simulink model "parallel_force_pos_control"  (R2020b)
settings: Solver=FixedStepAuto  StartTime=0.0  StopTime=10  FixedStep=Ts  RelTol=1e-3
undefined symbols (not defined in the file): dqi, fd, invMd, K, KD, KF, KI, KP, Md, myRobot, qi, xd, xr
settings Model: Creator=simon  LastModifiedBy=SimoneCremasco
settings SolverCC: ZeroCrossControl=DisableAll

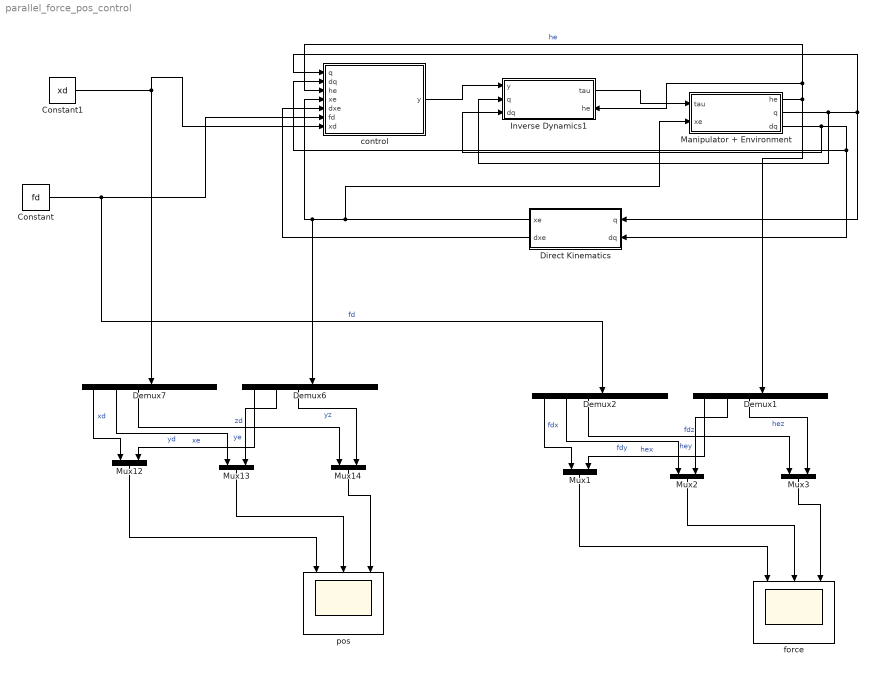
== system parallel_force_pos_control ==
  Constant : Constant  Value=fd
  Constant1 : Constant  Value=xd
  Demux{1..2,6..7} (4 alike) : Demux  Outputs=6
  Direct Kinematics : Subsystem
  Inverse Dynamics1 : Subsystem
      settings: PortSchema="{\"entries\":[{\"content\":{\"sides\":[{\"content\":{\"connectorIds\":[\"In1\",\"In2\",\"In3\"]},\"type\":\"ConnectorPlacement.EquallySpacedRectSide\",\"uuid\":\"75fd2aef-6636-4229-8361-fd4aaeafc71d\"},{\"content\":{\"connectorIds\":[\"Out1\",\"In4\"],\"side\":\"RIGHT\"},\"type\":\"ConnectorPlacement.EquallySpacedRectSide\",\"uuid\":\"1144ef1f-b296-4ded-9ece-76b41f9ae70a\"},{\"content\":{\"connectorIds\":[],\"side\":\"TOP\"},\"type\":\"ConnectorPlacement.EquallySpacedRectSide\",\"uuid\":\"a2369661-a37d-42fa-931f-950a2098898d\"},{\"content\":{\"connectorIds\":[],\"side\":\"BOTTOM\"},\"type\":\"ConnectorPlacement.EquallySpacedRectSide\",\"uuid\":\"99474d0a-a266-4b98-966c-e86b0204795e\"},{\"content\":{\"connectorIds\":[],\"side\":\"HIDDEN\"},\"type\":\"ConnectorPlacement.EquallySpacedRectSide\",\"uuid\":\"b2ea56db-8612-481b-8b10-64691d881ee0\"}]},\"type\":\"ConnectorPlacement.EquallySpacedConnector\",\"uuid\":\"7eb160dc-bfe8-4791-8ee2-e581093abb5e\"}],\"packageUris\":[\"http://schema.mathworks.com/mf0/Connector/R2020b\"],\"version\":\"1.0\"}"
  Manipulator + Environment : Subsystem
  Mux{1..3,12..14} (6 alike) : Mux  Inputs=2
  control : Subsystem
  force : Scope  NumInputPorts=3
  pos : Scope  NumInputPorts=3
  wires:
  Direct Kinematics/2(dxe) -> control/5(dxe)
  control/1(y) -> Inverse Dynamics1/1(y)
  Inverse Dynamics1/1(tau) -> Manipulator + Environment/1(tau)
  Manipulator + Environment/2(q) -> Inverse Dynamics1/2(q), Direct Kinematics/1(q), control/1(q)
  Manipulator + Environment/3(dq) -> Inverse Dynamics1/3(dq), Direct Kinematics/2(dq), control/2(dq)
  Manipulator + Environment/1(he) -> Inverse Dynamics1/4(he), control/3(he), Demux1/1  "he"
  Demux7/3 -> Mux14/1  "zd"
  Direct Kinematics/1(xe) -> Demux6/1, control/4(xe), Manipulator + Environment/2(xe)
  Constant/1 -> Demux2/1, control/6(fd)  "fd"
  Demux7/2 -> Mux13/1  "yd"
  Mux14/1 -> pos/3
  Demux7/1 -> Mux12/1  "xd"
  Demux6/2 -> Mux13/2  "ye"
  Demux6/1 -> Mux12/2  "xe"
  Demux6/3 -> Mux14/2  "yz"
  Mux12/1 -> pos/1
  Mux13/1 -> pos/2
  Constant1/1 -> control/7(xd), Demux7/1
  Mux2/1 -> force/2
  Mux1/1 -> force/1
  Mux3/1 -> force/3
  Demux2/3 -> Mux3/1  "fdz"
  Demux1/1 -> Mux1/2  "hex"
  Demux1/3 -> Mux3/2  "hez"
  Demux1/2 -> Mux2/2  "hey"
  Demux2/1 -> Mux1/1  "fdx"
  Demux2/2 -> Mux2/1  "fdy"

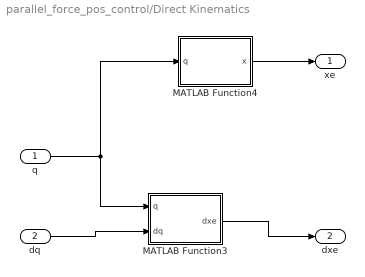
== system parallel_force_pos_control/Direct Kinematics ==
  q : Inport
  dq : Inport  Port=2
  MATLAB Function3 : MATLAB Function  TreatAsAtomicUnit=on
  MATLAB Function4 : MATLAB Function  TreatAsAtomicUnit=on
  xe : Outport
  dxe : Outport  Port=2
  wires:
  MATLAB Function3/1(dxe) -> dxe/1
  dq/1 -> MATLAB Function3/2(dq)
  q/1 -> MATLAB Function4/1(q), MATLAB Function3/1(q)
  MATLAB Function4/1(x) -> xe/1

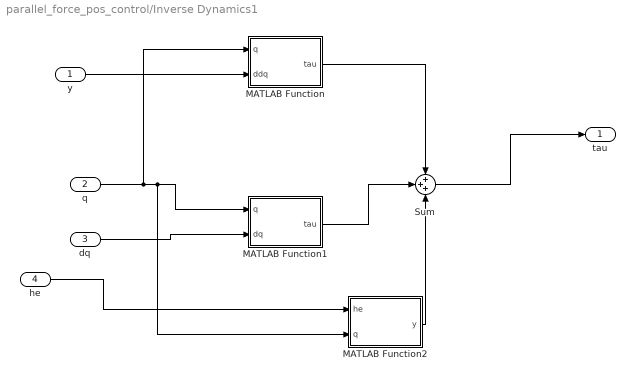
== system parallel_force_pos_control/Inverse Dynamics1 ==
  y : Inport
  q : Inport  Port=2
  dq : Inport  Port=3
  he : Inport  Port=4
  MATLAB Function : MATLAB Function  TreatAsAtomicUnit=on
  MATLAB Function1 : MATLAB Function  TreatAsAtomicUnit=on
  MATLAB Function2 : MATLAB Function  TreatAsAtomicUnit=on
  Sum : Sum  Inputs=+++
  tau : Outport
  wires:
  MATLAB Function1/1(tau) -> Sum/2
  MATLAB Function/1(tau) -> Sum/1
  y/1 -> MATLAB Function/2(ddq)
  dq/1 -> MATLAB Function1/2(dq)
  q/1 -> MATLAB Function/1(q), MATLAB Function2/2(q), MATLAB Function1/1(q)
  he/1 -> MATLAB Function2/1(he)
  MATLAB Function2/1(y) -> Sum/3
  Sum/1 -> tau/1

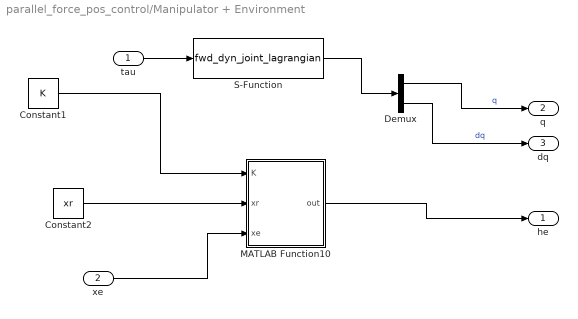
== system parallel_force_pos_control/Manipulator + Environment ==
  tau : Inport
  xe : Inport  Port=2
  Constant1 : Constant  Value=K
  Constant2 : Constant  Value=xr
  Demux : Demux  Outputs=2
  MATLAB Function10 : MATLAB Function  TreatAsAtomicUnit=on
  S-Function : S-Function  FunctionName=fwd_dyn_joint_lagrangian  Parameters=myRobot,qi,dqi  SFunctionDeploymentMode=off  EnableBusSupport=off
  he : Outport
  q : Outport  Port=2
  dq : Outport  Port=3
  wires:
  tau/1 -> S-Function/1
  Constant1/1 -> MATLAB Function10/1(K)
  Constant2/1 -> MATLAB Function10/2(xr)
  xe/1 -> MATLAB Function10/3(xe)
  S-Function/1 -> Demux/1
  Demux/1 -> q/1  "q"
  Demux/2 -> dq/1  "dq"
  MATLAB Function10/1(out) -> he/1

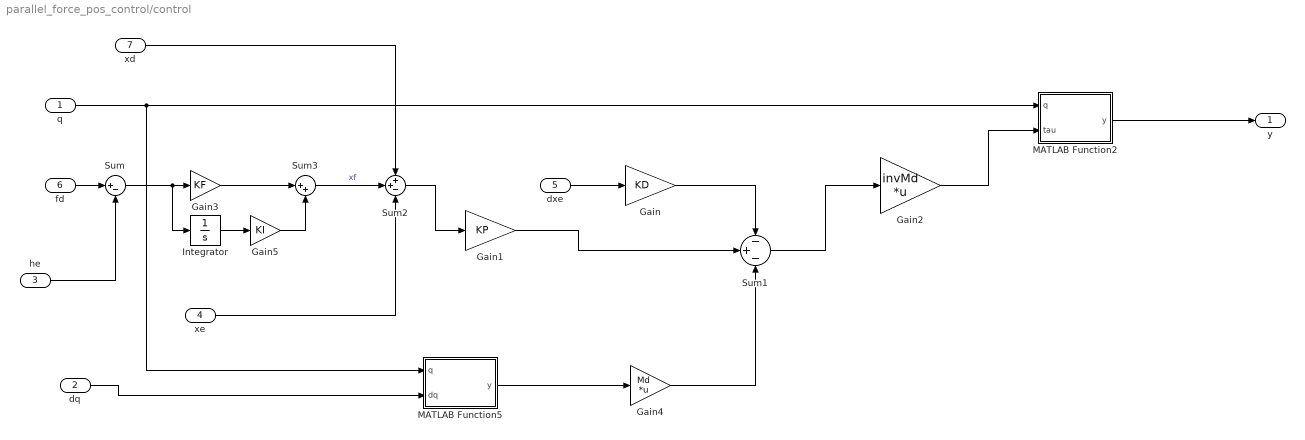
== system parallel_force_pos_control/control ==
  q : Inport
  dq : Inport  Port=2
  he : Inport  Port=3
  xe : Inport  Port=4
  dxe : Inport  Port=5
  fd : Inport  Port=6
  xd : Inport  Port=7
  Gain : Gain  Gain=KD
  Gain1 : Gain  Gain=KP
  Gain2 : Gain  Gain=invMd  Multiplication=Matrix(K*u)
  Gain3 : Gain  Gain=KF
  Gain4 : Gain  Gain=Md  Multiplication=Matrix(K*u)
  Gain5 : Gain  Gain=KI
  Integrator : Integrator
  MATLAB Function2 : MATLAB Function  TreatAsAtomicUnit=on
  MATLAB Function5 : MATLAB Function  TreatAsAtomicUnit=on
  Sum : Sum  Inputs=|+-
  Sum1 : Sum  Inputs=-+-
  Sum2 : Sum  Inputs=++-
  Sum3 : Sum  Inputs=|++
  y : Outport
  wires:
  MATLAB Function5/1(y) -> Gain4/1
  Gain2/1 -> MATLAB Function2/2(tau)
  MATLAB Function2/1(y) -> y/1
  dxe/1 -> Gain/1
  Sum1/1 -> Gain2/1
  Sum2/1 -> Gain1/1
  q/1 -> MATLAB Function5/1(q), MATLAB Function2/1(q)
  dq/1 -> MATLAB Function5/2(dq)
  Gain/1 -> Sum1/1
  Gain1/1 -> Sum1/2
  Gain4/1 -> Sum1/3
  fd/1 -> Sum/1
  Sum/1 -> Integrator/1, Gain3/1
  he/1 -> Sum/2
  Integrator/1 -> Gain5/1
  Gain3/1 -> Sum3/1
  Gain5/1 -> Sum3/2
  Sum3/1 -> Sum2/2  "xf"
  xe/1 -> Sum2/3
  xd/1 -> Sum2/1

== matlab function parallel_force_pos_control/Inverse Dynamics1/MATLAB Function ==
  data: q input size=3; tau output; ddq input size=3
function tau = B(q, ddq)

tau = getB(q)*ddq;

== matlab function parallel_force_pos_control/Inverse Dynamics1/MATLAB Function1 ==
  data: q input size=3; tau output; dq input size=3
function tau = n(q, dq)

tau = getN(q, dq);

== matlab function parallel_force_pos_control/Inverse Dynamics1/MATLAB Function2 ==
  data: he input; y output; q input
function y = fcn(he, q)
y = getJ(q)'*he;

== matlab function parallel_force_pos_control/control/MATLAB Function5 ==
  data: q input; y output; dq input
function y = dJa(q, dq)

y = getDiffJa(q)*dq;

== matlab function parallel_force_pos_control/Direct Kinematics/MATLAB Function3 ==
  data: q input; dxe output; dq input
function dxe = Ja(q, dq)

dxe = getJa(q)*dq;

== matlab function parallel_force_pos_control/control/MATLAB Function2 ==
  data: q input; y output; tau input
function y = invJ(q, tau)

y = getInvJ(q)*tau;

== matlab function parallel_force_pos_control/Direct Kinematics/MATLAB Function4 ==
  data: q input; x output
function x = k(q)

x = getK(q);

== matlab function parallel_force_pos_control/Manipulator + Environment/MATLAB Function10 ==
  data: K input; out output size=6; xr input; xe input size=6
function out = hde(K,xr, xe)
%consider the interaction only in z direction
out = zeros(6,1);
if xe(3) < xr(3)
    he = K*(xe-xr);
    out(3) = he(3);
end
